simulink model "noLoadmodel"  (R2021b)
settings: Solver=ode5  StartTime=0.0  StopTime=runT  FixedStep=dt  RelTol=1e-3
values from neighbouring files (symbols this model uses):
  Bm = bm * N * N    (= 2.601)    [noLoadInit.m]    (also in withLoadInit.m)
  den1c = [1, 2*zeta*wn, wn*wn]    [noLoadInit.m]    (also in withLoadInit.m)
  iMax = tauMax/Kt    (= 6.13841243116)    [noLoadInit.m]    (also in withLoadInit.m = 61.3841243116)
  Jm = jm * N * N    (= 0.023968215)    [noLoadInit.m]    (also in withLoadInit.m)
  Kt = 0.1118 * N    (= 5.7018)    [noLoadInit.m]    (also in withLoadInit.m)
  num1c = wn*wn    (= 1000000)    [noLoadInit.m]    (also in withLoadInit.m)
  tauMax = 35    [noLoadInit.m]    (also in withLoadInit.m = 350)
undefined symbols (not defined in the file or in its folder): stribeckFriction
libraries: simulink x2
settings Model: Creator=86135  LastModifiedBy=86135

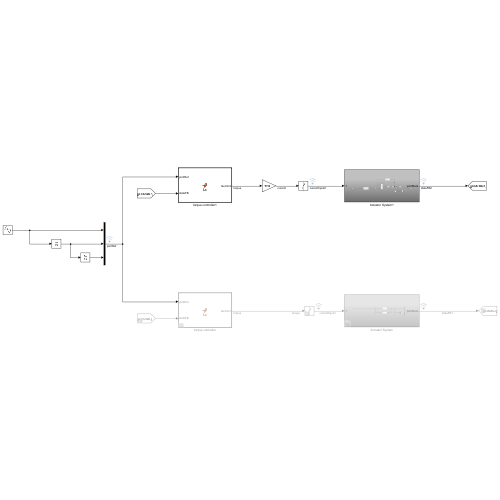
[thumbnail: Simulink's stored preview of the top-level diagram]
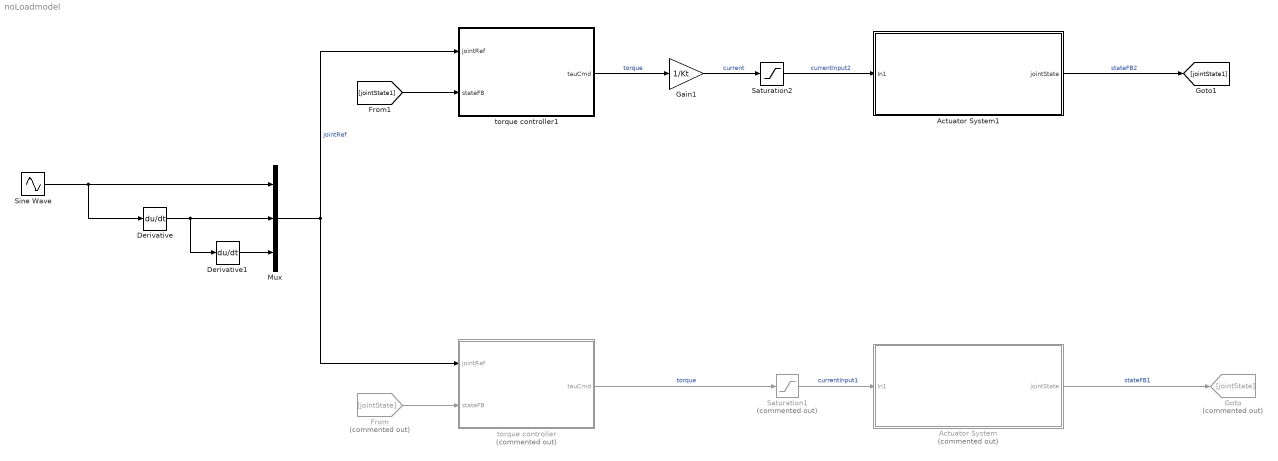
== system noLoadmodel ==
  Actuator System : Subsystem  Commented=on
  Actuator System1 : Subsystem
  Derivative : Derivative
  Derivative1 : Derivative
  From : From  Commented=on  GotoTag=jointState
  Gain1 : Gain  Gain=1/Kt
  Goto : Goto  Commented=on  GotoTag=jointState
  Mux : Mux  Inputs=3
  Saturation1 : Saturate  Commented=on  UpperLimit=tauMax  LowerLimit=-tauMax
  Saturation2 : Saturate  UpperLimit=iMax  LowerLimit=-iMax
  Sine Wave : Sin  Amplitude=3  Frequency=5  SampleTime=0
  torque controller : MATLAB Function  Commented=on  TreatAsAtomicUnit=on
  torque controller1 : MATLAB Function  TreatAsAtomicUnit=on
  wires:
  torque controller/1(tauCmd) -> Saturation1/1  "torque"
  Saturation1/1 -> Actuator System/1(In1)  "currentInput1"
  Actuator System/1(jointState) -> Goto/1  "stateFB1"
  From/1 -> torque controller/2(stateFB)
  Sine Wave/1 -> Mux/1, Derivative/1
  Derivative/1 -> Mux/2, Derivative1/1
  Mux/1 -> torque controller/1(jointRef), torque controller1/1(jointRef)  "jointRef"
  Derivative1/1 -> Mux/3
  Actuator System1/1(jointState) -> [jointState1]  "stateFB2"
  [jointState1] -> torque controller1/2(stateFB)
  torque controller1/1(tauCmd) -> Gain1/1  "torque"
  Gain1/1 -> Saturation2/1  "current"
  Saturation2/1 -> Actuator System1/1(In1)  "currentInput2"

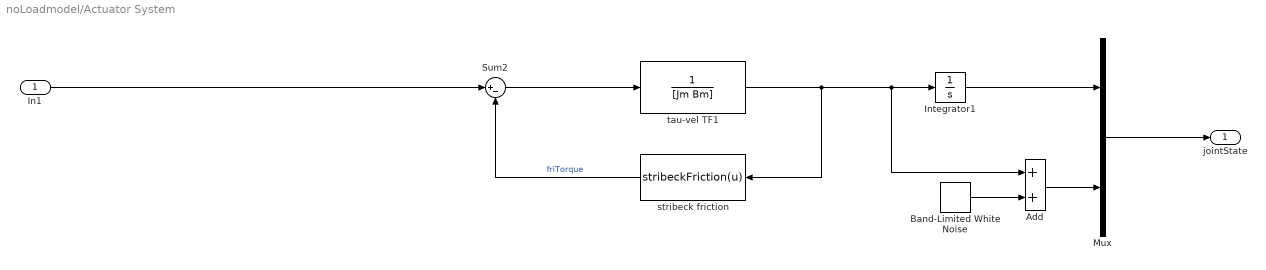
== system noLoadmodel/Actuator System ==
  In1 : Inport
  Add : Sum
  Band-Limited White Noise : simulink/Sources/Band-Limited White Noise  Cov=[0.00002]  Ts=0.001  seed=noiseSeedIndex
  Integrator1 : Integrator
  Mux : Mux  Inputs=2
  Sum2 : Sum  Inputs=|+-
  stribeck friction : MATLABFcn  MATLABFcn=stribeckFriction(u)
  tau-vel TF1 : TransferFcn  Denominator=[Jm Bm]
  jointState : Outport
  wires:
  tau-vel TF1/1 -> stribeck friction/1, Add/1, Integrator1/1
  stribeck friction/1 -> Sum2/2  "friTorque"
  Sum2/1 -> tau-vel TF1/1
  In1/1 -> Sum2/1
  Integrator1/1 -> Mux/1
  Add/1 -> Mux/2
  Mux/1 -> jointState/1
  Band-Limited White Noise/1 -> Add/2

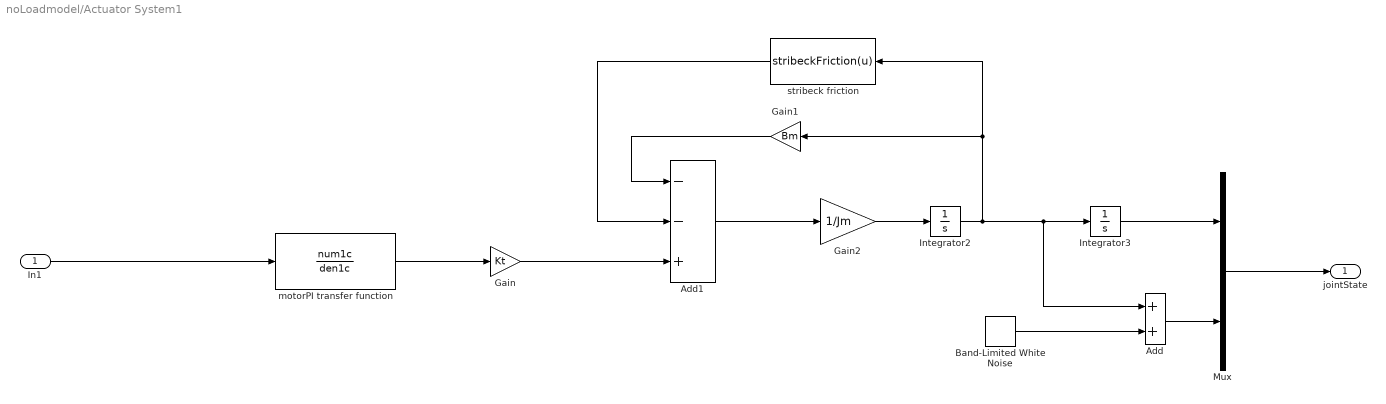
== system noLoadmodel/Actuator System1 ==
  In1 : Inport
  Add : Sum
  Add1 : Sum  Inputs=--+
  Band-Limited White Noise : simulink/Sources/Band-Limited White Noise  Cov=[0.00002]  Ts=0.001  seed=noiseSeedIndex
  Gain : Gain  Gain=Kt
  Gain1 : Gain  Gain=Bm
  Gain2 : Gain  Gain=1/Jm
  Integrator2 : Integrator
  Integrator3 : Integrator
  Mux : Mux  Inputs=2
  motorPI transfer function : TransferFcn  Numerator=num1c  Denominator=den1c
  stribeck friction : MATLABFcn  MATLABFcn=stribeckFriction(u)
  jointState : Outport
  wires:
  Gain1/1 -> Add1/1
  Add1/1 -> Gain2/1
  In1/1 -> motorPI transfer function/1
  Integrator2/1 -> Add/1, Integrator3/1, stribeck friction/1, Gain1/1
  Gain2/1 -> Integrator2/1
  Mux/1 -> jointState/1
  Add/1 -> Mux/2
  Gain/1 -> Add1/3
  stribeck friction/1 -> Add1/2
  Integrator3/1 -> Mux/1
  motorPI transfer function/1 -> Gain/1
  Band-Limited White Noise/1 -> Add/2

== matlab function noLoadmodel/torque controller1 ==
  data: jointRef input; tauCmd output; stateFB input; simPara parameter
function tauCmd = fcn(jointRef, stateFB, simPara)

qRef    = jointRef(1);
qdRef   = jointRef(2);
qddRef  = jointRef(3);
qFB     = stateFB(1);
qdFB    = stateFB(2);

Jm = simPara.Jm;
Bm = simPara.Bm;
kp = simPara.kp;
kd = simPara.kd;

friTorqueFFD = stribeckFriction(qdFB);

qError = qRef - qFB;
qdError = qdRef - qdFB;

feedbackTorque = kp * qError + kd * qdError;
feedforwardTorque = friTorqueFFD + Jm * qddRef + Bm * qdRef;
tauCmd = feedbackTorque + feedforwardTorque;
% tauCmd = feedforwardTorque;

== matlab function noLoadmodel/torque controller ==
  data: jointRef input; tauCmd output; stateFB input; simPara parameter
function tauCmd = fcn(jointRef, stateFB, simPara)

qRef    = jointRef(1);
qdRef   = jointRef(2);
qddRef  = jointRef(3);
qFB     = stateFB(1);
qdFB    = stateFB(2);

Jm = simPara.Jm;
Bm = simPara.Bm;
kp = simPara.kp;
kd = simPara.kd;

friTorqueFFD = stribeckFriction(qdFB);

qError = qRef - qFB;
qdError = qdRef - qdFB;

feedbackTorque = kp * qError + kd * qdError;
feedforwardTorque = friTorqueFFD + Jm * qddRef + Bm * qdRef;
tauCmd = feedbackTorque + feedforwardTorque;
% tauCmd = feedforwardTorque;
